simulink model "crane_sim_obs"  (R2016b)
settings: Solver=ode45  StartTime=0.0  StopTime=100  RelTol=1e-3  EnableMultiTasking=on
InitFcn:
  | param
undefined symbols (not defined in the file or in its folder): crane_ctrl, P
settings Model: Creator=beard  LastModifiedBy=Jacob
settings DataIOCC: LimitDataPoints=on  SaveFormat=Array  SignalLoggingSaveFormat=ModelDataLogs
settings OptimizationCC: ExpressionDepthLimit=2147483647  InitFltsAndDblsToZero=on  LifeSpan=inf
settings DebuggingCC: UnderspecifiedInitializationDetection=Classic  MergeDetectMultiDrivingBlocksExec=none  SolverPrmCheckMsg=warning  FcnCallInpInsideContextMsg=warning  StateNameClashWarn=warning  SFUnexpectedBacktrackingDiag=warning  SFNoUnconditionalDefaultTransitionDiag=warning  SFExecutionAtInitializationDiag=none
settings HardwareCC: ProdBitPerPointer=32  ProdBitPerSizeT=32  ProdBitPerPtrDiffT=32  ProdLargestAtomicFloat=None  ProdIntDivRoundTo=Undefined  ProdEndianess=Unspecified  ProdWordSize=32  ProdHWDeviceType=32-bit Generic
settings ModelReferenceCC: PropagateSignalLabelsOutOfModel=off
settings GRTTargetCC: TargetLangStandard=C89/C90 (ANSI)  GeneratePreprocessorConditionals=Disable all  CombineOutputUpdateFcns=off  GRTInterface=on
settings ConfigComp: CovMetricSettings=dw  CovHtmlReporting=on  CovSaveCumulativeToWorkspaceVar=on  CovSaveSingleToWorkspaceVar=on  CovExternalEMLEnable=off

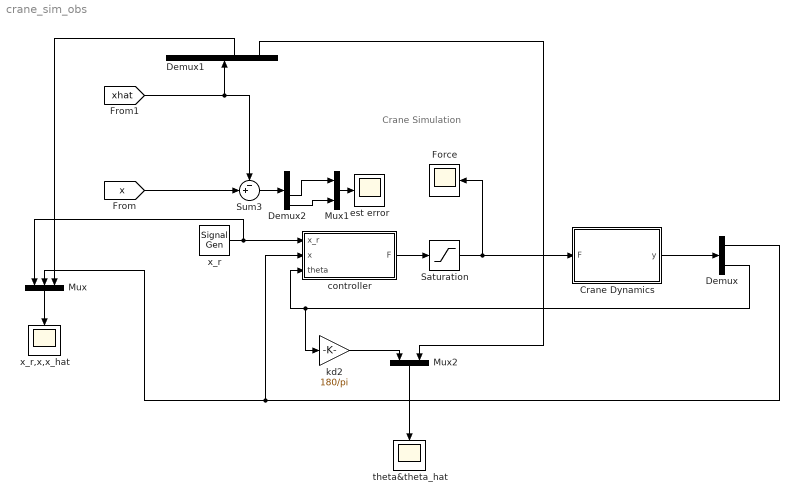
== system crane_sim_obs ==
  note: Crane Simulation
  Crane Dynamics : Subsystem
  Demux : Demux  Outputs=2
  Demux1 : Demux
  Demux2 : Demux
  Force : Scope
  Mux : Mux  Inputs=3
  Mux1 : Mux  Inputs=2
  Mux2 : Mux  Inputs=2
  Saturation : Saturate  UpperLimit=P.F_max  LowerLimit=-P.F_max
  Sum3 : Sum  Inputs=-+|
  controller : Subsystem
  est error : Scope
  kd2 : Gain  Gain=180/pi
  theta&theta_hat : Scope
  x_r : SignalGenerator  WaveForm=square  Amplitude=5  Frequency=.02
  x_r,x,x_hat : Scope
  wires:
  Crane Dynamics/1(y) -> Demux/1
  controller/1(F) -> Saturation/1
  x_r/1 -> controller/1(x_r), Mux/1
  Mux/1 -> x_r,x,x_hat/1
  Saturation/1 -> Crane Dynamics/1(F), Force/1
  Demux/1 -> controller/2("x "), Mux/2
  Demux/2 -> kd2/1, controller/3(theta)
  [xhat] -> Demux1/1, Sum3/1
  [x] -> Sum3/2
  Demux1/3 -> Mux/3
  Mux2/1 -> theta&theta_hat/1
  kd2/1 -> Mux2/1
  Demux1/4 -> Mux2/2
  Sum3/1 -> Demux2/1
  Mux1/1 -> est error/1
  Demux2/4 -> Mux1/2
  Demux2/3 -> Mux1/1

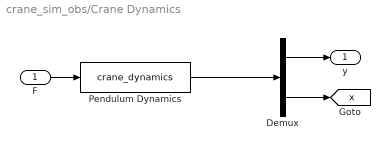
== system crane_sim_obs/Crane Dynamics ==
  F : Inport
  Demux : Demux  Outputs=[2;4]
  Pendulum Dynamics : S-Function  FunctionName=crane_dynamics  Parameters=P  SFunctionDeploymentMode=off  EnableBusSupport=off
  y : Outport
  tag scope: x=global
  wires:
  F/1 -> Pendulum Dynamics/1
  Demux/1 -> y/1
  Pendulum Dynamics/1 -> Demux/1
  Demux/2 -> [x]

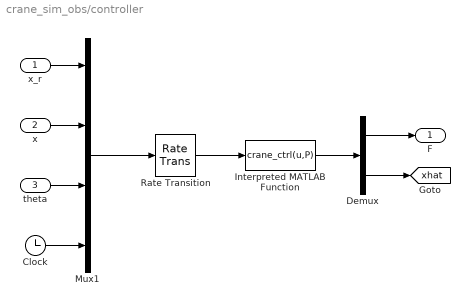
== system crane_sim_obs/controller ==
  x_r : Inport
  "x " : Inport  Port=2
  theta : Inport  Port=3
  Clock : Clock
  Demux : Demux  Outputs=[1;4]
  Interpreted MATLAB Function : MATLABFcn  MATLABFcn=crane_ctrl(u,P)  OutputDimensions=1+4
  Mux1 : Mux
  Rate Transition : RateTransition  OutPortSampleTime=P.Ts
  F : Outport
  tag scope: xhat=global
  wires:
  Mux1/1 -> Rate Transition/1
  x_r/1 -> Mux1/1
  Clock/1 -> Mux1/4
  Rate Transition/1 -> Interpreted MATLAB Function/1
  theta/1 -> Mux1/3
  "x "/1 -> Mux1/2
  Interpreted MATLAB Function/1 -> Demux/1
  Demux/1 -> F/1
  Demux/2 -> [xhat]
